simulink model "ControlSystem_Refactorization"  (R2025a)
settings: Solver=FixedStepAuto  StartTime=0.0  StopTime=inf  FixedStep=1e-4  RelTol=1e-3
PostLoadFcn:
  | clear;
  | load_system('ControlSystem_Refactorization');
  | evalin('base', 'run("inicializarBuses.m")');
values from neighbouring files (symbols this model uses):
  actuadorBus = arrayfun(@(x) Simulink.Bus.createMATLABStruct(actuadorBusInfo.busName, x), actuador)    [inicializarBuses.m]
undefined symbols (not defined in the file or in its folder): Configuracion, Controlador, Estado, EstadoValvula, ModoControl, National_Instruments, ParametroControl, PCIe
libraries: simulink x11, sldrtlib x5
(part 2 of 2)

== system ControlSystem_Refactorization/untitledPanel6 ==
  Combo Box : ComboBox  Tag=HiddenForWebPanel  PanelInfo="{\"height\":31,\"left\":66,\"panelId\":\"panelId-25e449ab-1693-49df-8bc5-822e2c020e76\",\"top\":325,\"type\":\"panelChild\",\"version\":\"2019b\",\"width\":200,\"zIndex\":1500010}"  LabelPosition=Hide  SelectedLabel=Actuador 1
  Lamp : LampBlock  Tag=HiddenForWebPanel  PanelInfo="{\"height\":105,\"left\":120,\"panelId\":\"panelId-25e449ab-1693-49df-8bc5-822e2c020e76\",\"top\":101,\"type\":\"panelChild\",\"version\":\"2019b\",\"width\":114,\"zIndex\":1500012}"  LabelPosition=Hide  DefaultColor=[192.0, 192.0, 192.0]
  Rotary Switch : RotarySwitchBlock  Tag=HiddenForWebPanel  PanelInfo="{\"height\":125,\"left\":10,\"panelId\":\"panelId-25e449ab-1693-49df-8bc5-822e2c020e76\",\"top\":416,\"type\":\"panelChild\",\"version\":\"2019b\",\"width\":156,\"zIndex\":1500002}"  LabelPosition=Hide  UseEnumeratedDataType=on  EnumeratedDataType=EstadoValvula
  Rotary Switch1 : RotarySwitchBlock  Tag=HiddenForWebPanel  PanelInfo="{\"height\":125,\"left\":188,\"panelId\":\"panelId-25e449ab-1693-49df-8bc5-822e2c020e76\",\"top\":417,\"type\":\"panelChild\",\"version\":\"2019b\",\"width\":156,\"zIndex\":1500006}"  LabelPosition=Hide  UseEnumeratedDataType=on  EnumeratedDataType=EstadoValvula
  Rotary Switch2 : RotarySwitchBlock  Tag=HiddenForWebPanel  PanelInfo="{\"height\":125,\"left\":15,\"panelId\":\"panelId-25e449ab-1693-49df-8bc5-822e2c020e76\",\"top\":584,\"type\":\"panelChild\",\"version\":\"2019b\",\"width\":156,\"zIndex\":1500008}"  LabelPosition=Hide  UseEnumeratedDataType=on  EnumeratedDataType=EstadoValvula
  Rotary Switch3 : RotarySwitchBlock  Tag=HiddenForWebPanel  PanelInfo="{\"height\":125,\"left\":188,\"panelId\":\"panelId-25e449ab-1693-49df-8bc5-822e2c020e76\",\"top\":583,\"type\":\"panelChild\",\"version\":\"2019b\",\"width\":156,\"zIndex\":1500004}"  LabelPosition=Hide  UseEnumeratedDataType=on  EnumeratedDataType=EstadoValvula
  panelInfo : PanelWebBlock  Tag=HiddenForWebPanel  PanelInfo="{\"compacted\":false,\"height\":768,\"isActiveTab\":false,\"labels\":{\"label1570808903\":{\"deleted\":false,\"left\":107,\"settings\":{\"backgroundColor\":\"rgba(0, 0, 0, 0)\",\"bold\":true,\"font\":\"Arial\",\"fontColor\":\"black\",\"fontSize\":1,\"italicized\":false,\"underlined\":false},\"text\":\"FLUJO DE AIRE\",\"top\":389},\"label1904916882\":{\"deleted\":false,\"left\":48,\"settings\":{\"backgroundColor\":\"rgba(0, 0, 0, 0)\",\"bold\":true,\"font\":\"Arial\",\"fontColor\":\"black\",\"fontSize\":1,\"italicized\":false,\"underlined\":false},\"text\":\"ACTUADOR DE REFERENCIA\",\"top\":294},\"label4554094127\":{\"deleted\":false,\"left\":59,\"settings\":{\"backgroundColor\":\"rgba(0, 0, 0, 0)\",\"bold\":false,\"font\":\"Arial\",\"fontColor\":\"black\",\"fontSize\":0.9,\"italicized\":false,\"underlined\":false},\"text\":\"Actuador 3\",\"top\":713},\"label5544201829\":{\"deleted\":false,\"left\":55,\"settings\":{\"backgroundColor\":\"rgba(0, 0, 0, 0)\",\"bold\":false,\"font\":\"Arial\",\"fontColor\":\"black\",\"fontSize\":0.9,\"italicized\":false,\"underlined\":false},\"text\":\"Actuador 1\",\"top\":550},\"label7257437999\":{\"deleted\":false,\"left\":244,\"settings\":{\"backgroundColor\":\"rgba(0, 0, 0, 0)\",\"bold\":false,\"font\":\"Arial\",\"fontColor\":\"black\",\"fontSize\":0.9,\"italicized\":false,\"underlined\":false},\"text\":\"Actuador 4\",\"top\":718},\"label8713368904\":{\"deleted\":false,\"left\":93,\"settings\":{\"backgroundColor\":\"rgba(0, 0, 0, 0)\",\"bold\":true,\"font\":\"Arial\",\"fontColor\":\"black\",\"fontSize\":1.1,\"italicized\":false,\"underlined\":false},\"text\":\"CONTROL MANUAL\",\"top\":42},\"label9472504070\":{\"deleted\":false,\"left\":233,\"settings\":{\"backgroundColor\":\"rgba(0, 0, 0, 0)\",\"bold\":false,\"font\":\"Arial\",\"fontColor\":\"black\",\"fontSize\":0.9,\"italicized\":false,\"underlined\":false},\"text\":\"Actuador 2\",\"top\":552}},\"left\":854,\"name\":\"Control Manual\",\"panelId\":\"panelId-25e449ab-1693-49df-8bc5-822e2c020e76\",\"tabIndex\":0,\"tabbedSetId\":\"tabbedSet0009314149\",\"top\":26,\"type\":\"panel\",\"version\":\"2019b\",\"visible\":false,\"width\":362,\"zIndex\":1500012}"  PanelSnapshot=<binary blob, 86348 chars, not shown>

== system ControlSystem_Refactorization/untitledPanel8 ==
  Lamp : LampBlock  Tag=HiddenForWebPanel  PanelInfo="{\"height\":70,\"left\":26,\"panelId\":\"panelId-b53b3ba2-c29a-424b-9a86-7082199ec354\",\"top\":32,\"type\":\"panelChild\",\"version\":\"2019b\",\"width\":75,\"zIndex\":1500002}"  LabelPosition=Hide  DefaultColor=[192.0, 192.0, 192.0]
  Slider Switch1 : SliderSwitchBlock  Tag=HiddenForWebPanel  PanelInfo="{\"height\":35,\"left\":19,\"panelId\":\"panelId-b53b3ba2-c29a-424b-9a86-7082199ec354\",\"top\":109,\"type\":\"panelChild\",\"version\":\"2019b\",\"width\":89,\"zIndex\":1500004}"  LabelPosition=Hide
  panelInfo : PanelWebBlock  Tag=HiddenForWebPanel  PanelInfo="{\"compacted\":false,\"height\":151,\"isActiveTab\":true,\"labels\":{\"label0400441507\":{\"deleted\":false,\"left\":15,\"settings\":{\"backgroundColor\":\"rgba(0, 0, 0, 0)\",\"bold\":true,\"font\":\"Arial\",\"fontColor\":\"black\",\"fontSize\":0.93,\"italicized\":false,\"underlined\":false},\"text\":\"SIMULACIÓN\",\"top\":11}},\"left\":322,\"name\":\"Simulacion\",\"panelId\":\"panelId-b53b3ba2-c29a-424b-9a86-7082199ec354\",\"tabIndex\":0,\"tabbedSetId\":\"tabbedSet4721076845\",\"top\":27,\"type\":\"panel\",\"version\":\"2019b\",\"visible\":true,\"width\":129,\"zIndex\":1500020}"  PanelSnapshot=<binary blob, 15904 chars, not shown>

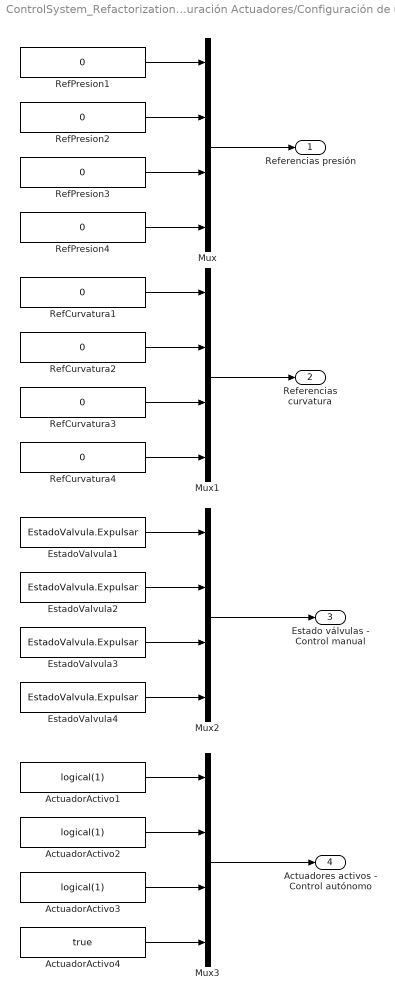
== system ControlSystem_Refactorization/Configuración Actuadores/Configuración de usuario ==
  ActuadorActivo1 : Constant  Value=logical(1)
  ActuadorActivo2 : Constant  Value=logical(1)
  ActuadorActivo3 : Constant  Value=logical(1)
  ActuadorActivo4 : Constant  Value=true
  EstadoValvula{1..4} (4 alike) : Constant  Value=EstadoValvula.Expulsar
  Mux{,1..3} (4 alike) : Mux
  RefCurvatura{1..4} (4 alike) : Constant  Value=0
  RefPresion{1..4} (4 alike) : Constant  Value=0
  Referencias presión : Outport
  Referencias curvatura : Outport  Port=2
  Estado válvulas - Control manual : Outport  Port=3
  Actuadores activos - Control autónomo : Outport  Port=4
  wires:
  RefPresion2/1 -> Mux/2
  RefPresion1/1 -> Mux/1
  RefPresion3/1 -> Mux/3
  RefPresion4/1 -> Mux/4
  RefCurvatura3/1 -> Mux1/3
  RefCurvatura2/1 -> Mux1/2
  RefCurvatura1/1 -> Mux1/1
  RefCurvatura4/1 -> Mux1/4
  EstadoValvula3/1 -> Mux2/3
  EstadoValvula2/1 -> Mux2/2
  EstadoValvula1/1 -> Mux2/1
  EstadoValvula4/1 -> Mux2/4
  Mux/1 -> Referencias presión/1
  Mux1/1 -> Referencias curvatura/1
  Mux2/1 -> Estado válvulas - Control manual/1
  ActuadorActivo4/1 -> Mux3/4
  ActuadorActivo3/1 -> Mux3/3
  ActuadorActivo1/1 -> Mux3/1
  ActuadorActivo2/1 -> Mux3/2
  Mux3/1 -> Actuadores activos - Control autónomo/1

== system ControlSystem_Refactorization/Configuración Actuadores/For Each Subsystem ==
  Bus : Inport  Partition=on  PartitionDimension=1  PartitionWidth=1  PartitionOffset=0
  Referencias de presión : Inport  Port=2  Partition=on  PartitionDimension=1  PartitionWidth=1  PartitionOffset=0
  Referencias de curvatura : Inport  Port=3  Partition=on  PartitionDimension=1  PartitionWidth=1  PartitionOffset=0
  Estado válvulas - Control manual : Inport  Port=4  Partition=on  PartitionDimension=1  PartitionWidth=1  PartitionOffset=0
  Actuadores activos - Control autónomo : Inport  Port=5  Partition=on  PartitionDimension=1  PartitionWidth=1  PartitionOffset=0
  Bus Assignment3 : BusAssignment  AssignedSignals=Configuracion.Global.activo,Configuracion.ControlManual.estadoValvula,Configuracion.Global.Referencia.presion,Configuracion.Global.Referencia.curvatura
  For Each : ForEach  DisableCoverage=on
  Out1 : Outport  ConcatenationDimension=1
  wires:
  Bus Assignment3/1 -> Out1/1
  Bus/1 -> Bus Assignment3/1
  Referencias de curvatura/1 -> Bus Assignment3/5
  Referencias de presión/1 -> Bus Assignment3/4
  Estado válvulas - Control manual/1 -> Bus Assignment3/3
  Actuadores activos - Control autónomo/1 -> Bus Assignment3/2

== system ControlSystem_Refactorization/Configuración Sistema/Configuración de usuario ==
  Constant : Constant  Value=ModoControl(1)
  Constant1 : Constant  Value=ParametroControl(0)
  Constant2 : Constant
  Constant4 : Constant
  Constant5 : Constant  Value=0.01
  Constant6 : Constant  Value=0.01
  Constant7 : Constant  Value=0.001
  Constant8 : Constant  Value=0.001
  Constant9 : Constant  Value=0.01
  Modo de control : Outport
  Parámetro de control : Outport  Port=2
  Simulación activa : Outport  Port=3
  Actuador seleccionado : Outport  Port=4
  Tolerancia Presión Estacionaria : Outport  Port=5
  Tolerancia Presión Derivativa : Outport  Port=6
  Tolerancia Curvatura Estacionaria : Outport  Port=7
  Tolerancia Curvatura Derivativa : Outport  Port=8
  Tolerancia Equilibrio Presiones : Outport  Port=9
  wires:
  Constant/1 -> Modo de control/1
  Constant1/1 -> Parámetro de control/1
  Constant2/1 -> Simulación activa/1
  Constant4/1 -> Actuador seleccionado/1
  Constant5/1 -> Tolerancia Presión Estacionaria/1
  Constant6/1 -> Tolerancia Presión Derivativa/1
  Constant7/1 -> Tolerancia Curvatura Estacionaria/1
  Constant8/1 -> Tolerancia Curvatura Derivativa/1
  Constant9/1 -> Tolerancia Equilibrio Presiones/1

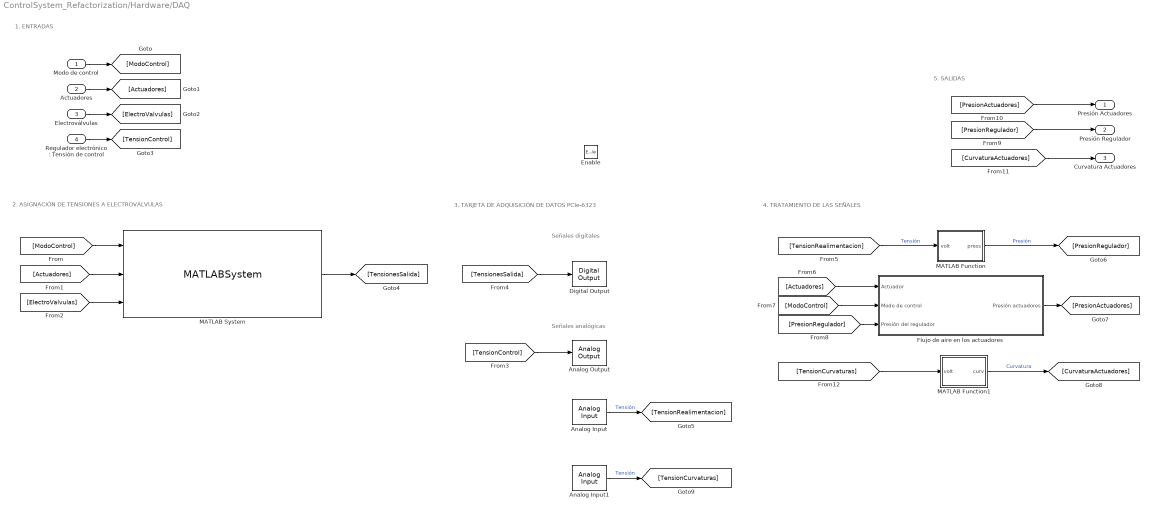
== system ControlSystem_Refactorization/Hardware/DAQ ==
  note: 5. SALIDAS
  note: 4. TRATAMIENTO DE LAS SEÑALES
  note: 1. ENTRADAS
  note: 2. ASIGNACIÓN DE TENSIONES A ELECTROVÁLVULAS
  note: 3. TARJETA DE ADQUISICIÓN DE DATOS
      | PCIe-6323
  note: Señales analógicas
  note: Señales digitales
  Modo de control : Inport
  Actuadores : Inport  Port=2
  Electroválvulas : Inport  Port=3
  Regulador electrónico: Tensión de control : Inport  Port=4
  Enable : EnablePort
  Analog Input : sldrtlib/Analog Input  SampleTime=0.1  MaxMissedTicks=10  ShowMissedTicks=off  YieldWhenWaiting=off  DrvName=National_Instruments/PCIe-6323  DrvAddress=4294967295  DrvOptions=[1 31 0 0 0 0 0]  Channels=1  RangeMode=1  VoltRange=1  DataType=1
      settings: AttributesFormatString=National Instruments\nPCIe-6323 [auto]
  Analog Input1 : sldrtlib/Analog Input  SampleTime=0.1  MaxMissedTicks=10  ShowMissedTicks=off  YieldWhenWaiting=off  DrvName=National_Instruments/PCIe-6323  DrvAddress=4294967295  DrvOptions=[1 31 0 0 0 0 0]  Channels=[2 3 4 5]  RangeMode=1  VoltRange=1  DataType=1
      settings: AttributesFormatString=National Instruments\nPCIe-6323 [auto]
  Analog Output : sldrtlib/Analog Output  SampleTime=0.1  MaxMissedTicks=10  ShowMissedTicks=off  YieldWhenWaiting=off  DrvName=National_Instruments/PCIe-6323  DrvAddress=4294967295  DrvOptions=[1 31 0 0 0 0 0]  Channels=1  RangeMode=1  VoltRange=1  InitialValue=[]  FinalValue=[]
      settings: AttributesFormatString=National Instruments\nPCIe-6323 [auto]
  Digital Output : sldrtlib/Digital Output  SampleTime=0.1  MaxMissedTicks=10  ShowMissedTicks=off  YieldWhenWaiting=off  DrvName=National_Instruments/PCIe-6323  DrvAddress=4294967295  DrvOptions=[0 255 0 0 0 0 0]  Channels=[1 2 3 4 5 6 7 8]  BitMode=1  InitialValue=[]  FinalValue=[]
      settings: AttributesFormatString=National Instruments\nPCIe-6323 [auto]
  Flujo de aire en los actuadores : Subsystem  TreatAsAtomicUnit=on
  MATLAB Function : MATLAB Function  TreatAsAtomicUnit=on
  MATLAB Function1 : MATLAB Function  TreatAsAtomicUnit=on
  MATLAB System : MATLABSystem  System=selectElectrovalvesVoltage  SimulateUsing=Code generation
      mask Type: selectElectrovalvesVoltage
  Presión Actuadores : Outport
  Presión Regulador : Outport  Port=2
  Curvatura Actuadores : Outport  Port=3
  wires:
  Modo de control/1 -> [ModoControl]
  [ModoControl] -> MATLAB System/1
  Actuadores/1 -> [Actuadores]
  [Actuadores] -> MATLAB System/2
  Electroválvulas/1 -> [ElectroValvulas]
  [ElectroValvulas] -> MATLAB System/3
  Regulador electrónico: Tensión de control/1 -> [TensionControl]
  [TensionControl] -> Analog Output/1
  MATLAB System/1 -> [TensionesSalida]
  [TensionesSalida] -> Digital Output/1
  [TensionRealimentacion] -> MATLAB Function/1(volt)  "Tensión"
  Flujo de aire en los actuadores/1(Presión actuadores) -> [PresionActuadores]
  [Actuadores] -> Flujo de aire en los actuadores/1(Actuador)
  [ModoControl] -> Flujo de aire en los actuadores/2(Modo de control)
  MATLAB Function/1(press) -> [PresionRegulador]  "Presión"
  [PresionRegulador] -> Flujo de aire en los actuadores/3(Presión del regulador)
  [TensionCurvaturas] -> MATLAB Function1/1(volt)
  [CurvaturaActuadores] -> Curvatura Actuadores/1
  [PresionActuadores] -> Presión Actuadores/1
  [PresionRegulador] -> Presión Regulador/1
  Analog Input/1 -> [TensionRealimentacion]  "Tensión"
  Analog Input1/1 -> [TensionCurvaturas]  "Tensión"
  MATLAB Function1/1(curv) -> [CurvaturaActuadores]  "Curvatura"

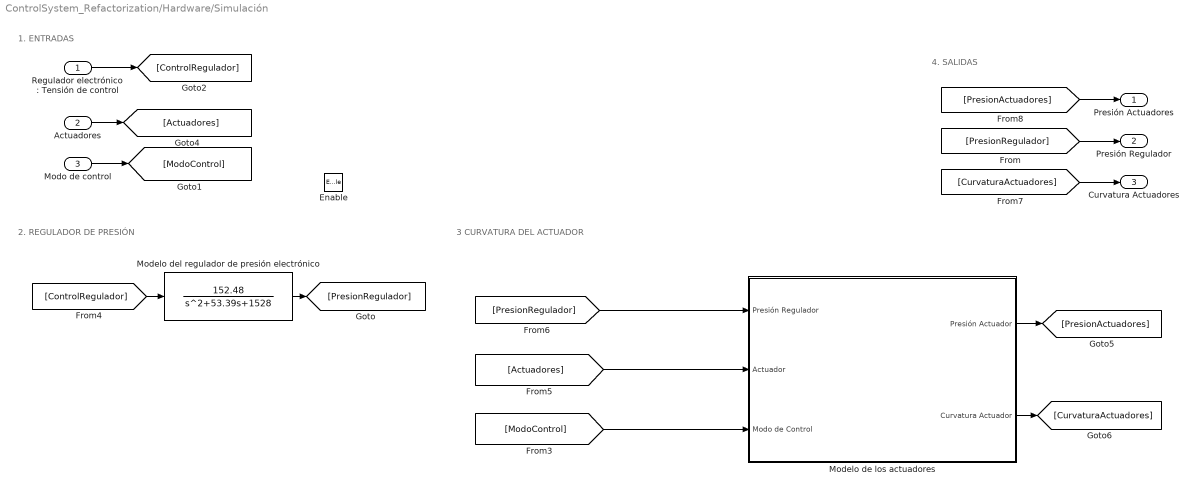
== system ControlSystem_Refactorization/Hardware/Simulación ==
  note: 4. SALIDAS
  note: 3 CURVATURA DEL ACTUADOR
  note: 2. REGULADOR DE PRESIÓN
  note: 1. ENTRADAS
  Regulador electrónico: Tensión de control : Inport
  Actuadores : Inport  Port=2
  Modo de control : Inport  Port=3
  Enable : EnablePort
  Modelo de los actuadores : Subsystem  TreatAsAtomicUnit=on
  Modelo del regulador de presión electrónico : TransferFcn  Numerator=[0 0 152.48]  Denominator=[1 53.39 1528]
  Presión Actuadores : Outport
  Presión Regulador : Outport  Port=2
  Curvatura Actuadores : Outport  Port=3
  wires:
  Regulador electrónico: Tensión de control/1 -> [ControlRegulador]
  Modo de control/1 -> [ModoControl]
  [ModoControl] -> Modelo de los actuadores/3(Modo de Control)
  Modelo del regulador de presión electrónico/1 -> [PresionRegulador]
  [ControlRegulador] -> Modelo del regulador de presión electrónico/1
  [Actuadores] -> Modelo de los actuadores/2(Actuador)
  Modelo de los actuadores/1(Presión Actuador) -> [PresionActuadores]
  Modelo de los actuadores/2(Curvatura Actuador) -> [CurvaturaActuadores]
  [PresionRegulador] -> Presión Regulador/1
  [CurvaturaActuadores] -> Curvatura Actuadores/1
  [PresionActuadores] -> Presión Actuadores/1
  [PresionRegulador] -> Modelo de los actuadores/1(Presión Regulador)
  Actuadores/1 -> [Actuadores]

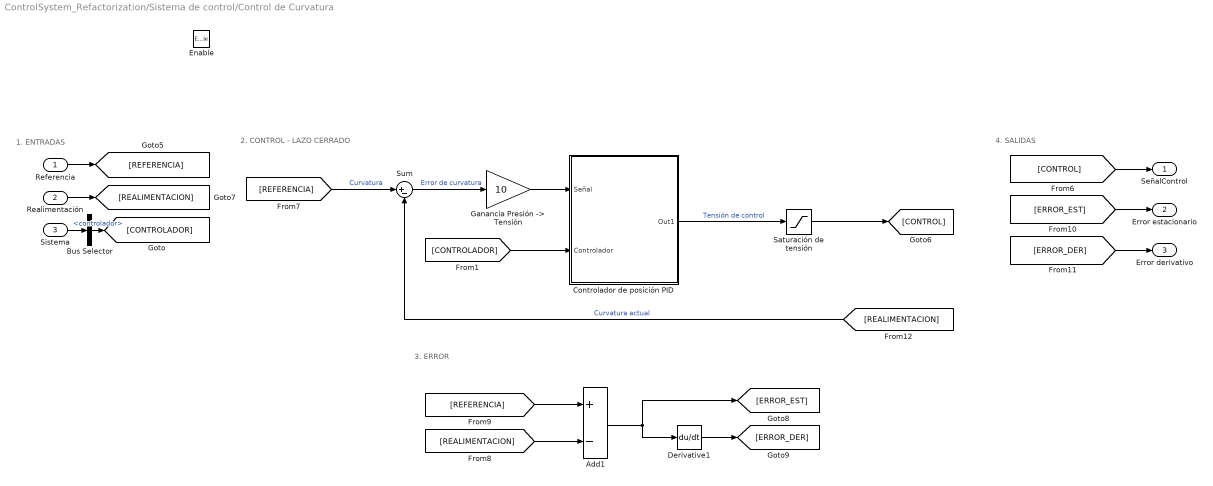
== system ControlSystem_Refactorization/Sistema de control/Control de Curvatura ==
  note: 4. SALIDAS
  note: 3. ERROR
  note: 2. CONTROL - LAZO CERRADO
  note: 1. ENTRADAS
  Referencia : Inport
  Realimentación : Inport  Port=2
  Sistema : Inport  Port=3
  Enable : EnablePort  StatesWhenEnabling=reset  ZeroCross=off
  Add1 : Sum  Inputs=+-
  Bus Selector : BusSelector  OutputSignals=Configuracion.Global.controlador
  Controlador de posición PID : Subsystem  TreatAsAtomicUnit=on
  Derivative1 : Derivative
  "Ganancia Presión -> Tensión" : Gain  Gain=10
  Saturación de tensión : Saturate  UpperLimit=10  LowerLimit=0  ZeroCross=off
  Sum : Sum  Inputs=|+-
  SeñalControl : Outport
  Error estacionario : Outport  Port=2
  Error derivativo : Outport  Port=3
  wires:
  [ERROR_EST] -> Error estacionario/1
  [CONTROL] -> SeñalControl/1
  Realimentación/1 -> [REALIMENTACION]
  [REFERENCIA] -> Sum/1  "Curvatura"
  [REFERENCIA] -> Add1/1
  [ERROR_DER] -> Error derivativo/1
  [REALIMENTACION] -> Add1/2
  [REALIMENTACION] -> Sum/2  "Curvatura actual"
  Add1/1 -> [ERROR_EST], Derivative1/1
  Referencia/1 -> [REFERENCIA]
  Sum/1 -> "Ganancia Presión -> Tensión"/1  "Error de curvatura"
  Derivative1/1 -> [ERROR_DER]
  Saturación de tensión/1 -> [CONTROL]
  Controlador de posición PID/1(Out1) -> Saturación de tensión/1  "Tensión de control"
  "Ganancia Presión -> Tensión"/1 -> Controlador de posición PID/1(Señal)
  Sistema/1 -> Bus Selector/1
  Bus Selector/1 -> [CONTROLADOR]  "<controlador>"
  [CONTROLADOR] -> Controlador de posición PID/2(Controlador)

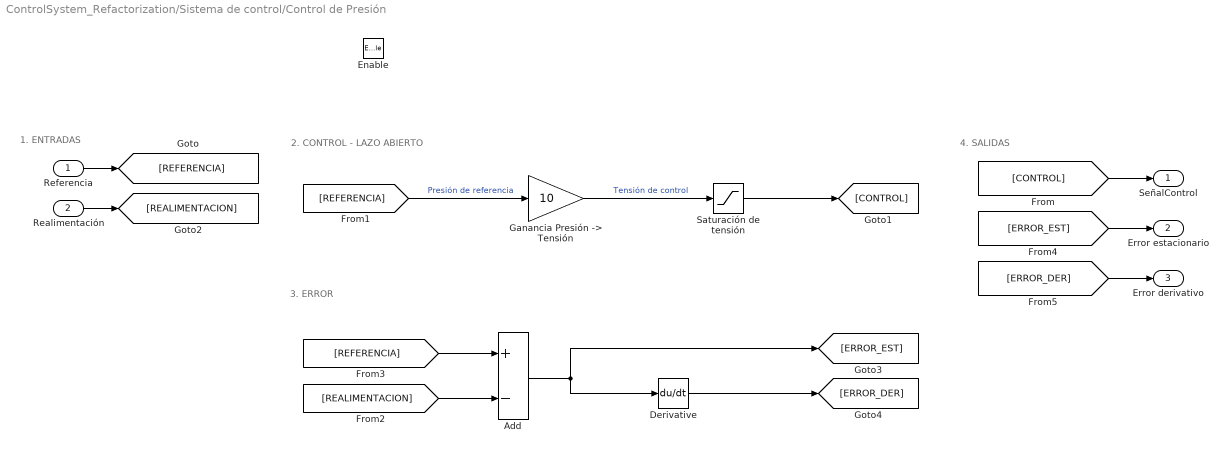
== system ControlSystem_Refactorization/Sistema de control/Control de Presión ==
  note: 1. ENTRADAS
  note: 4. SALIDAS
  note: 3. ERROR
  note: 2. CONTROL - LAZO ABIERTO
  Referencia : Inport
  Realimentación : Inport  Port=2
  Enable : EnablePort  StatesWhenEnabling=reset
  Add : Sum  Inputs=+-
  Derivative : Derivative
  "Ganancia Presión -> Tensión" : Gain  Gain=10
  Saturación de tensión : Saturate  UpperLimit=10  LowerLimit=0
  SeñalControl : Outport
  Error estacionario : Outport  Port=2
  Error derivativo : Outport  Port=3
  wires:
  Realimentación/1 -> [REALIMENTACION]
  [ERROR_DER] -> Error derivativo/1
  [ERROR_EST] -> Error estacionario/1
  [REALIMENTACION] -> Add/2
  Derivative/1 -> [ERROR_DER]
  Referencia/1 -> [REFERENCIA]
  "Ganancia Presión -> Tensión"/1 -> Saturación de tensión/1  "Tensión de control"
  [CONTROL] -> SeñalControl/1
  Add/1 -> [ERROR_EST], Derivative/1
  [REFERENCIA] -> "Ganancia Presión -> Tensión"/1  "Presión de referencia"
  [REFERENCIA] -> Add/1
  Saturación de tensión/1 -> [CONTROL]

== system ControlSystem_Refactorization/Visualización de datos en interfaz/DATOS DE ACTUADORES ==
  actuadores : Inport  Partition=on  PartitionDimension=1  PartitionWidth=1  PartitionOffset=0
  Bus Selector : BusSelector  OutputSignals=Estado.Realimentacion.presion,Estado.Realimentacion.curvatura,Estado.ControlAutomatico.actuadorPosicionado
  For Each : ForEach  DisableCoverage=on
  Presión actuadores : Outport  ConcatenationDimension=1
  Curvatura actuadores : Outport  Port=2  ConcatenationDimension=1
  Actuadores posicionados : Outport  Port=3  ConcatenationDimension=1
  wires:
  actuadores/1 -> Bus Selector/1
  Bus Selector/1 -> Presión actuadores/1  "<presion>"
  Bus Selector/2 -> Curvatura actuadores/1  "<curvatura>"
  Bus Selector/3 -> Actuadores posicionados/1  "<actuadorPosicionado>"

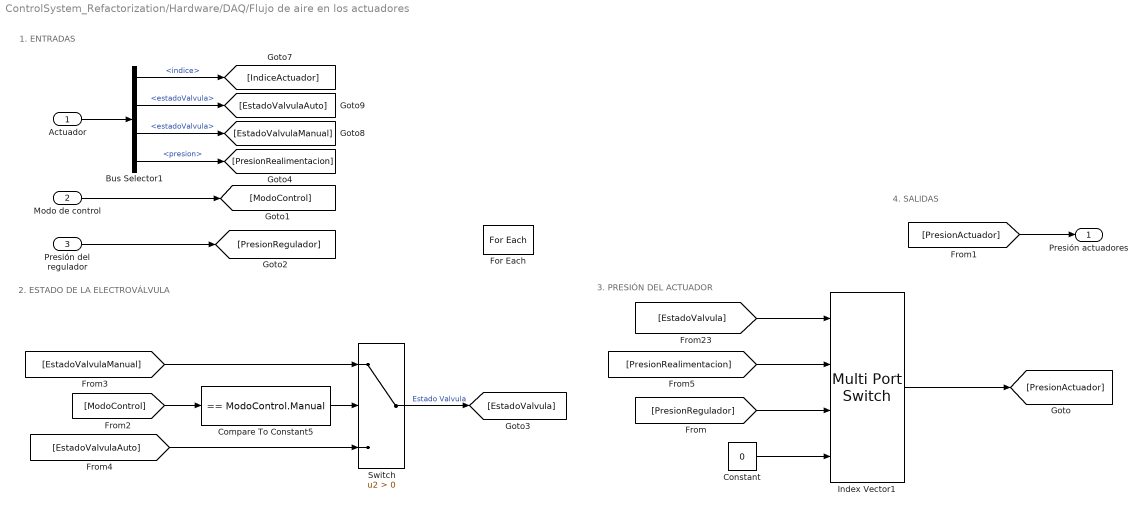
== system ControlSystem_Refactorization/Hardware/DAQ/Flujo de aire en los actuadores ==
  note: 4. SALIDAS
  note: 3. PRESIÓN DEL ACTUADOR
  note: 1. ENTRADAS
  note: 2. ESTADO DE LA ELECTROVÁLVULA
  Actuador : Inport  Partition=on  PartitionDimension=1  PartitionWidth=1  PartitionOffset=0
  Modo de control : Inport  Port=2
  Presión del regulador : Inport  Port=3
  Bus Selector1 : BusSelector  OutputSignals=Configuracion.Global.indice,Estado.ControlAutomatico.estadoValvula,Configuracion.ControlManual.estadoValvula,Estado.Realimentacion.presion
  Compare To Constant5 : simulink/Logic and Bit Operations/Compare To Constant  relop===  const=ModoControl.Manual  OutDataTypeStr=boolean
  Constant : Constant  Value=0
  For Each : ForEach  DisableCoverage=on
  Index Vector1 : MultiPortSwitch  DataPortOrder=Specify indices  DataPortIndices={EstadoValvula.Bloquear, EstadoValvula.Inyectar, EstadoValvula.Expulsar}  SaturateOnIntegerOverflow=off  InputSameDT=off
  Switch : Switch  Criteria=u2 > Threshold  SaturateOnIntegerOverflow=off  InputSameDT=off
  Presión actuadores : Outport  ConcatenationDimension=1
  wires:
  [EstadoValvula] -> Index Vector1/1
  Constant/1 -> Index Vector1/4
  [PresionRegulador] -> Index Vector1/3
  Index Vector1/1 -> [PresionActuador]
  Bus Selector1/1 -> [IndiceActuador]  "<indice>"
  Bus Selector1/3 -> [EstadoValvulaManual]  "<estadoValvula>"
  Actuador/1 -> Bus Selector1/1
  Bus Selector1/2 -> [EstadoValvulaAuto]  "<estadoValvula>"
  Modo de control/1 -> [ModoControl]
  Presión del regulador/1 -> [PresionRegulador]
  [PresionActuador] -> Presión actuadores/1
  [EstadoValvulaAuto] -> Switch/3
  Switch/1 -> [EstadoValvula]  "Estado Valvula"
  Compare To Constant5/1 -> Switch/2
  [ModoControl] -> Compare To Constant5/1
  [EstadoValvulaManual] -> Switch/1
  Bus Selector1/4 -> [PresionRealimentacion]  "<presion>"
  [PresionRealimentacion] -> Index Vector1/2

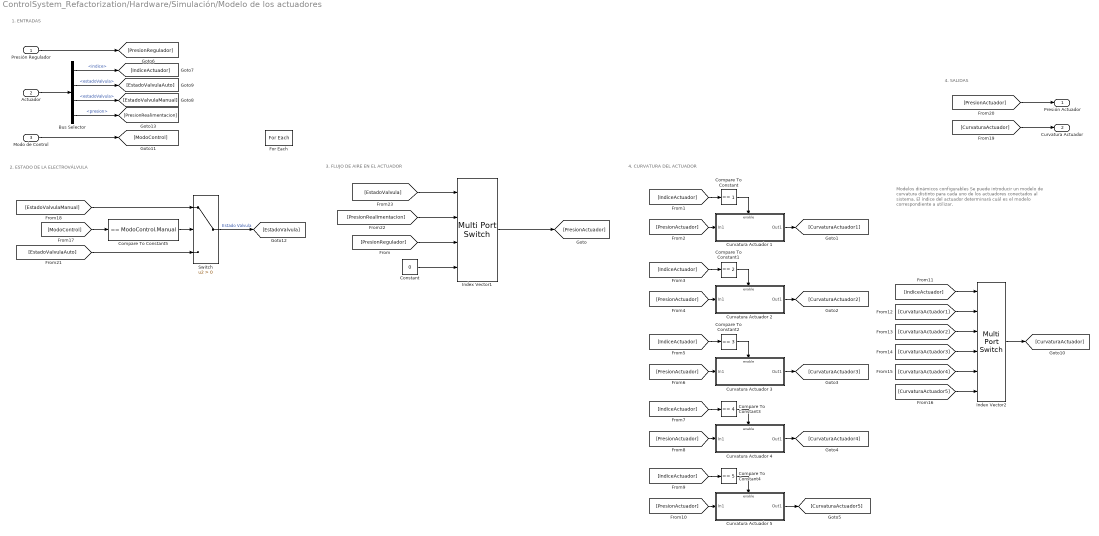
== system ControlSystem_Refactorization/Hardware/Simulación/Modelo de los actuadores ==
  note: 2. ESTADO DE LA ELECTROVÁLVULA
  note: Modelos dinámicos configurables
      |
      | Se puede introducir un modelo de curvatura distinto para cada uno de los actuadores conectados al sistema.
      |
      | El índice del actuador determinará cuál es el modelo correspondiente a utilizar.
  note: 1. ENTRADAS
  note: 4. CURVATURA DEL ACTUADOR
  note: 3. FLUJO DE AIRE EN EL ACTUADOR
  note: 4. SALIDAS
  Presión Regulador : Inport
  Actuador : Inport  Port=2  Partition=on  PartitionDimension=1  PartitionWidth=1  PartitionOffset=0
  Modo de Control : Inport  Port=3
  Bus Selector : BusSelector  OutputSignals=Configuracion.Global.indice,Estado.ControlAutomatico.estadoValvula,Configuracion.ControlManual.estadoValvula,Estado.Realimentacion.presion
  Compare To Constant : simulink/Logic and Bit Operations/Compare To Constant  relop===  const=1  OutDataTypeStr=boolean
  Compare To Constant1 : simulink/Logic and Bit Operations/Compare To Constant  relop===  const=2  OutDataTypeStr=boolean
  Compare To Constant2 : simulink/Logic and Bit Operations/Compare To Constant  relop===  const=3  OutDataTypeStr=boolean
  Compare To Constant3 : simulink/Logic and Bit Operations/Compare To Constant  relop===  const=4  OutDataTypeStr=boolean
  Compare To Constant4 : simulink/Logic and Bit Operations/Compare To Constant  relop===  const=5  OutDataTypeStr=boolean
  Compare To Constant5 : simulink/Logic and Bit Operations/Compare To Constant  relop===  const=ModoControl.Manual  OutDataTypeStr=boolean
  Constant : Constant  Value=0
  Curvatura Actuador 1 : Subsystem  TreatAsAtomicUnit=on
  Curvatura Actuador 2 : Subsystem  TreatAsAtomicUnit=on
  Curvatura Actuador 3 : Subsystem  TreatAsAtomicUnit=on
  Curvatura Actuador 4 : Subsystem  TreatAsAtomicUnit=on
  Curvatura Actuador 5 : Subsystem  TreatAsAtomicUnit=on
  For Each : ForEach  DisableCoverage=on
  Index Vector1 : MultiPortSwitch  DataPortOrder=Specify indices  DataPortIndices={EstadoValvula.Bloquear, EstadoValvula.Inyectar, EstadoValvula.Expulsar}  SaturateOnIntegerOverflow=off  InputSameDT=off
  Index Vector2 : MultiPortSwitch  Inputs=5  SaturateOnIntegerOverflow=off  InputSameDT=off
  Switch : Switch  Criteria=u2 > Threshold  SaturateOnIntegerOverflow=off  InputSameDT=off
  Presión Actuador : Outport  ConcatenationDimension=1
  Curvatura Actuador : Outport  Port=2  ConcatenationDimension=1
  wires:
  Presión Regulador/1 -> [PresionRegulador]
  [PresionRegulador] -> Index Vector1/3
  Constant/1 -> Index Vector1/4
  Index Vector1/1 -> [PresionActuador]
  Compare To Constant/1 -> Curvatura Actuador 1/Enable
  [IndiceActuador] -> Compare To Constant/1
  [PresionActuador] -> Curvatura Actuador 1/1(In1)
  Compare To Constant1/1 -> Curvatura Actuador 2/Enable
  [IndiceActuador] -> Compare To Constant1/1
  [PresionActuador] -> Curvatura Actuador 2/1(In1)
  Compare To Constant2/1 -> Curvatura Actuador 3/Enable
  [IndiceActuador] -> Compare To Constant2/1
  [PresionActuador] -> Curvatura Actuador 3/1(In1)
  Compare To Constant3/1 -> Curvatura Actuador 4/Enable
  [IndiceActuador] -> Compare To Constant3/1
  [PresionActuador] -> Curvatura Actuador 4/1(In1)
  Compare To Constant4/1 -> Curvatura Actuador 5/Enable
  [IndiceActuador] -> Compare To Constant4/1
  [PresionActuador] -> Curvatura Actuador 5/1(In1)
  [IndiceActuador] -> Index Vector2/1
  [CurvaturaActuador2] -> Index Vector2/3
  [CurvaturaActuador1] -> Index Vector2/2
  [CurvaturaActuador5] -> Index Vector2/6
  [CurvaturaActuador4] -> Index Vector2/5
  [CurvaturaActuador3] -> Index Vector2/4
  Curvatura Actuador 1/1(Out1) -> [CurvaturaActuador1]
  Curvatura Actuador 2/1(Out1) -> [CurvaturaActuador2]
  Curvatura Actuador 3/1(Out1) -> [CurvaturaActuador3]
  Curvatura Actuador 4/1(Out1) -> [CurvaturaActuador4]
  Curvatura Actuador 5/1(Out1) -> [CurvaturaActuador5]
  Index Vector2/1 -> [CurvaturaActuador]
  [CurvaturaActuador] -> Curvatura Actuador/1
  [PresionActuador] -> Presión Actuador/1
  Actuador/1 -> Bus Selector/1
  Bus Selector/1 -> [IndiceActuador]  "<indice>"
  Bus Selector/2 -> [EstadoValvulaAuto]  "<estadoValvula>"
  Bus Selector/3 -> [EstadoValvulaManual]  "<estadoValvula>"
  Modo de Control/1 -> [ModoControl]
  [EstadoValvulaAuto] -> Switch/3
  Switch/1 -> [EstadoValvula]  "Estado Valvula"
  [EstadoValvula] -> Index Vector1/1
  Compare To Constant5/1 -> Switch/2
  [EstadoValvulaManual] -> Switch/1
  [ModoControl] -> Compare To Constant5/1
  Bus Selector/4 -> [PresionRealimentacion]  "<presion>"
  [PresionRealimentacion] -> Index Vector1/2

== system ControlSystem_Refactorization/Sistema de control/Control de Curvatura/Controlador de posición PID ==
  note: Esta señal reinicia el valor del control integral cada vez que se cambia de controlador
      | o actuador
  note: Proporcional
  note: Integral
  note: Derivativo
  Señal : Inport
  Controlador : Inport  Port=2
  Add : Sum  Inputs=+++
  Compare To Constant : simulink/Logic and Bit Operations/Compare To Constant  relop===  const=Controlador.Curvatura  OutDataTypeStr=boolean
  Derivative : Derivative
  Gain : Gain  Gain=65
  Gain1 : Gain  Gain=233.3
  Gain2 : Gain  Gain=1.25
  Integrator : Integrator  ExternalReset=either  UpperSaturationLimit=10  LowerSaturationLimit=-10  ZeroCross=off
  Out1 : Outport
  wires:
  Señal/1 -> Gain/1, Gain1/1, Gain2/1
  Add/1 -> Out1/1  "control"
  Gain/1 -> Add/1
  Gain1/1 -> Integrator/1
  Gain2/1 -> Derivative/1
  Integrator/1 -> Add/2
  Derivative/1 -> Add/3
  Controlador/1 -> Compare To Constant/1
  Compare To Constant/1 -> [CONTROL_ACTIVO]
  [CONTROL_ACTIVO] -> Integrator/2

== system ControlSystem_Refactorization/Hardware/Simulación/Modelo de los actuadores/Curvatura Actuador 1 ==
  In1 : Inport
  Enable : EnablePort
  Modelo de curvatura del actuador : TransferFcn  Numerator=[995.3 1595 424.3 7.903]  Denominator=[1 1.141e04 7.488e04 7.239e04 1.423e04 143]
  Out1 : Outport
  wires:
  In1/1 -> Modelo de curvatura del actuador/1
  Modelo de curvatura del actuador/1 -> Out1/1  "CurvAct"

== system ControlSystem_Refactorization/Hardware/Simulación/Modelo de los actuadores/Curvatura Actuador 2 ==
  In1 : Inport
  Enable : EnablePort
  Modelo de curvatura del actuador1 : TransferFcn  Numerator=[995.3 1595 424.3 7.903]  Denominator=[1 1.141e04 7.488e04 7.239e04 1.423e04 143]
  Out1 : Outport
  wires:
  In1/1 -> Modelo de curvatura del actuador1/1
  Modelo de curvatura del actuador1/1 -> Out1/1  "CurvAct"

== system ControlSystem_Refactorization/Hardware/Simulación/Modelo de los actuadores/Curvatura Actuador 3 ==
  In1 : Inport
  Enable : EnablePort
  Modelo de curvatura del actuador1 : TransferFcn  Numerator=[995.3 1595 424.3 7.903]  Denominator=[1 1.141e04 7.488e04 7.239e04 1.423e04 143]
  Out1 : Outport
  wires:
  In1/1 -> Modelo de curvatura del actuador1/1
  Modelo de curvatura del actuador1/1 -> Out1/1  "CurvAct"

== system ControlSystem_Refactorization/Hardware/Simulación/Modelo de los actuadores/Curvatura Actuador 4 ==
  In1 : Inport
  Enable : EnablePort
  Modelo de curvatura del actuador1 : TransferFcn  Numerator=[995.3 1595 424.3 7.903]  Denominator=[1 1.141e04 7.488e04 7.239e04 1.423e04 143]
  Out1 : Outport
  wires:
  In1/1 -> Modelo de curvatura del actuador1/1
  Modelo de curvatura del actuador1/1 -> Out1/1  "CurvAct"

== system ControlSystem_Refactorization/Hardware/Simulación/Modelo de los actuadores/Curvatura Actuador 5 ==
  In1 : Inport
  Enable : EnablePort
  Modelo de curvatura del actuador : TransferFcn  Numerator=[995.3 1595 424.3 7.903]  Denominator=[1 1.141e04 7.488e04 7.239e04 1.423e04 143]
  Out1 : Outport
  wires:
  In1/1 -> Modelo de curvatura del actuador/1
  Modelo de curvatura del actuador/1 -> Out1/1  "CurvAct"

== matlab function ControlSystem_Refactorization/Hardware/DAQ/MATLAB Function ==
  data: volt input; press output
function press = volt2press(volt)
% Obtiene la presión actual de salida del regulador electrónico a partir de
% su señal de tensión medida

%% Parámetros del regulador de presión
% Fijos
voltMin = 0.9836; % Tensión a presión = 0 bar
voltMax = 1.7976; % Tensión a presión = barMax
% Configurables
barMax = 1; % Presión a tensión = voltMax

%% Relación Tensión/Presión
% Relación V/P
k = (voltMax-voltMin)/barMax;
% Medida de presión
press = (volt-voltMin)/k;

== matlab function ControlSystem_Refactorization/Hardware/DAQ/MATLAB Function1 ==
  data: volt input; curv output
function curv = volt2curv(volt)
% Obtiene la curvatura actual de un actuador a partir de la tensión medida
% por su sensor de curvatura

%% Parámetros de curvatura
% V = A*C + B
A = [62.6723, 63.6333, 63.6685, 62.6754]';
B = [2.3357, 2.3916, 2.4152, 2.4385]';

%% Relación Tensión/Curvatura
% C = (V-B)/A
curv = (volt-B)./A;
